simulink subsystem "KF_gyrostellar"  (R2021a)
settings: Solver=VariableStepAuto  StartTime=0.0  StopTime=10.0  RelTol=1e-3
undefined symbols (not defined in the file): bias_gyro_init, gyro_bias_init, init_align_error, magnitude
libraries: dspmtrx3 x1, sharedtransform x1
settings Model: Creator=Laura  LastModifiedBy=jmher

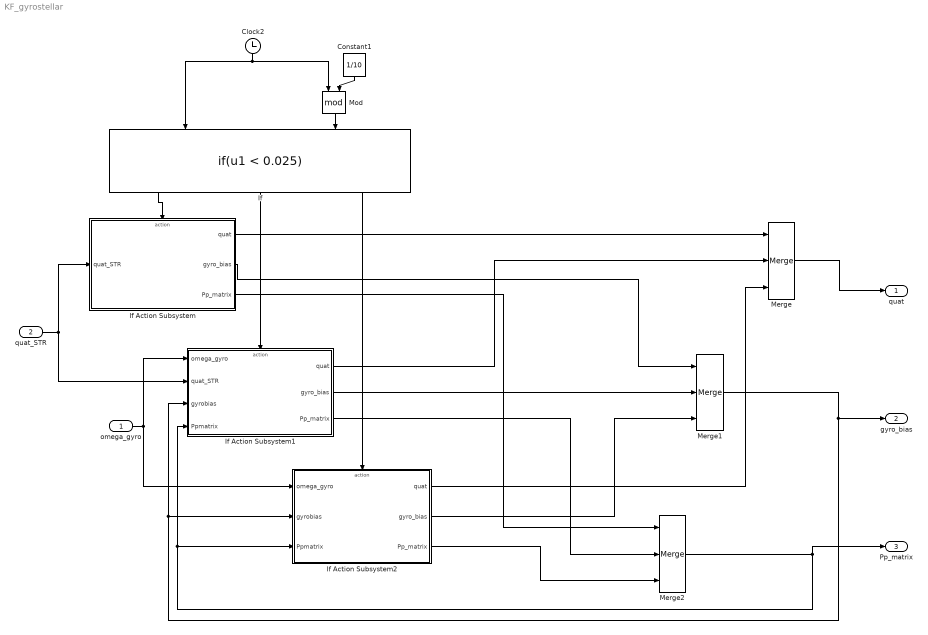
== system KF_gyrostellar ==
  omega_gyro : Inport
  quat_STR : Inport  Port=2
  Clock2 : Clock
  Constant1 : Constant  Value=1/10
  If : If  NumInputs=2  IfExpression=u1 < 0.025  ElseIfExpressions=u2 == 0
  If Action Subsystem : Subsystem  TreatAsAtomicUnit=on
  If Action Subsystem1 : Subsystem  TreatAsAtomicUnit=on
  If Action Subsystem2 : Subsystem  TreatAsAtomicUnit=on
  Merge : Merge  Inputs=3
  Merge1 : Merge  Inputs=3
  Merge2 : Merge  Inputs=3
  Mod : Math  Operator=mod  SaturateOnIntegerOverflow=on
  quat : Outport
  gyro_bias : Outport  Port=2
  Pp_matrix : Outport  Port=3
  wires:
  Clock2/1 -> Mod/1, If/1
  Constant1/1 -> Mod/2
  Mod/1 -> If/2
  If Action Subsystem2/1(quat) -> Merge/3
  Merge/1 -> quat/1
  If Action Subsystem/1(quat) -> Merge/1
  If Action Subsystem/2(gyro_bias) -> Merge1/1
  If Action Subsystem1/2(gyro_bias) -> Merge1/2
  If Action Subsystem2/2(gyro_bias) -> Merge1/3
  If Action Subsystem2/3(Pp_matrix) -> Merge2/3
  If Action Subsystem/3(Pp_matrix) -> Merge2/1
  If Action Subsystem1/3(Pp_matrix) -> Merge2/2
  Merge1/1 -> gyro_bias/1, If Action Subsystem1/3(gyrobias), If Action Subsystem2/2(gyrobias)
  quat_STR/1 -> If Action Subsystem1/2(quat_STR), If Action Subsystem/1(quat_STR)
  Merge2/1 -> Pp_matrix/1, If Action Subsystem2/3(Ppmatrix), If Action Subsystem1/4(Ppmatrix)
  If/1 -> If Action Subsystem/Action
  omega_gyro/1 -> If Action Subsystem2/1(omega_gyro), If Action Subsystem1/1(omega_gyro)
  If/2 -> If Action Subsystem1/Action
  If Action Subsystem1/1(quat) -> Merge/2
  If/3 -> If Action Subsystem2/Action

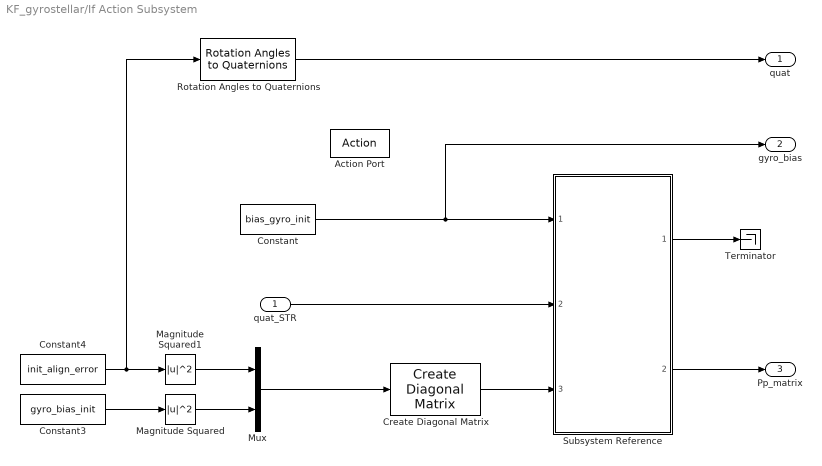
== system KF_gyrostellar/If Action Subsystem ==
  quat_STR : Inport
  Action Port : ActionPort  ActionPortLabel=if(u1 < 0.025)
  Constant : Constant  Value=bias_gyro_init
  Constant3 : Constant  Value=gyro_bias_init
  Constant4 : Constant  Value=init_align_error
  Create Diagonal Matrix : dspmtrx3/Create Diagonal Matrix
      settings: SourceProductBaseCode=DS
  Magnitude Squared : Math  Operator=magnitude^2  SaturateOnIntegerOverflow=on
  Magnitude Squared1 : Math  Operator=magnitude^2  SaturateOnIntegerOverflow=on
  Mux : Mux  Inputs=2
  Rotation Angles to Quaternions : sharedtransform/Rotation Angles to Quaternions  rotationOrder=ZYX  aMode=aMode
      settings: SourceProductBaseCode=AE,PW,DR,MT,UV,VE
  Subsystem Reference : Subsystem  ReferencedSubsystem=KF_update
  Terminator : Terminator
  quat : Outport
  gyro_bias : Outport  Port=2
  Pp_matrix : Outport  Port=3
  wires:
  Magnitude Squared1/1 -> Mux/1
  Constant3/1 -> Magnitude Squared/1
  Mux/1 -> Create Diagonal Matrix/1
  Constant/1 -> gyro_bias/1, Subsystem Reference/1
  Create Diagonal Matrix/1 -> Subsystem Reference/3
  Subsystem Reference/2 -> Pp_matrix/1
  Rotation Angles to Quaternions/1 -> quat/1
  Constant4/1 -> Rotation Angles to Quaternions/1, Magnitude Squared1/1
  Magnitude Squared/1 -> Mux/2
  Subsystem Reference/1 -> Terminator/1
  quat_STR/1 -> Subsystem Reference/2

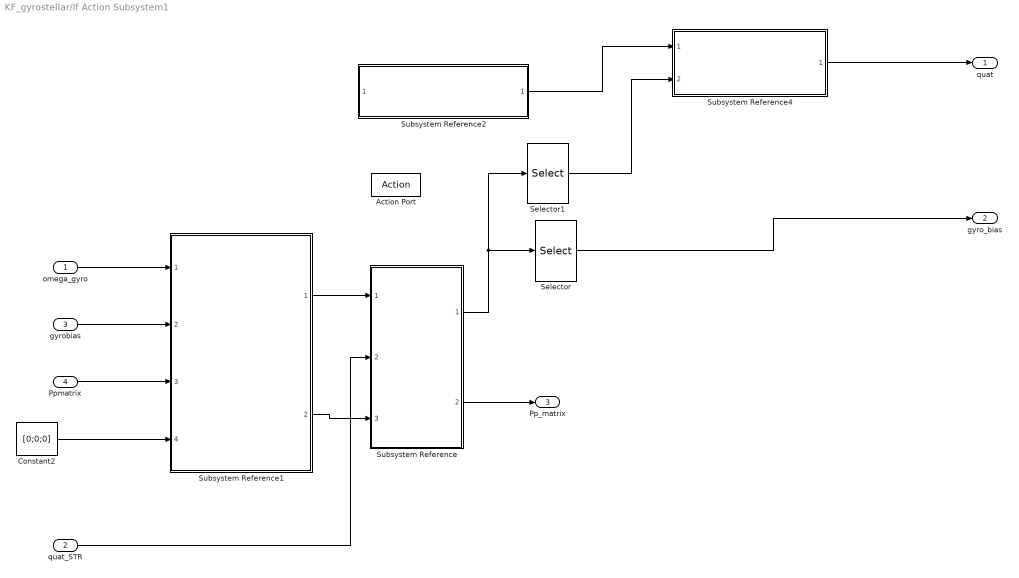
== system KF_gyrostellar/If Action Subsystem1 ==
  omega_gyro : Inport
  quat_STR : Inport  Port=2
  gyrobias : Inport  Port=3
  Ppmatrix : Inport  Port=4
  Action Port : ActionPort  ActionPortLabel=elseif(u2 == 0 )
  Constant2 : Constant  Value=[0;0;0]
  Selector : Selector  InputPortWidth=6  IndexOptions=Index vector (dialog)  Indices=[4 5 6]  OutputSizes=1
  Selector1 : Selector  InputPortWidth=6  IndexOptions=Index vector (dialog)  Indices=[1 2 3]  OutputSizes=1
  Subsystem Reference : Subsystem  ReferencedSubsystem=KF_update
  Subsystem Reference1 : Subsystem  ReferencedSubsystem=KF_prediction
  Subsystem Reference2 : Subsystem  ReferencedSubsystem=GyroIntegrator
  Subsystem Reference4 : Subsystem  ReferencedSubsystem=QuaternionUpdate
  quat : Outport
  gyro_bias : Outport  Port=2
  Pp_matrix : Outport  Port=3
  wires:
  Selector/1 -> gyro_bias/1
  quat_STR/1 -> Subsystem Reference/2
  omega_gyro/1 -> Subsystem Reference1/1
  gyrobias/1 -> Subsystem Reference1/2
  Subsystem Reference/2 -> Pp_matrix/1
  Constant2/1 -> Subsystem Reference1/4
  Subsystem Reference1/1 -> Subsystem Reference/1
  Subsystem Reference4/1 -> quat/1
  Subsystem Reference2/1 -> Subsystem Reference4/1
  Selector1/1 -> Subsystem Reference4/2
  Ppmatrix/1 -> Subsystem Reference1/3
  Subsystem Reference1/2 -> Subsystem Reference/3
  Subsystem Reference/1 -> Selector1/1, Selector/1

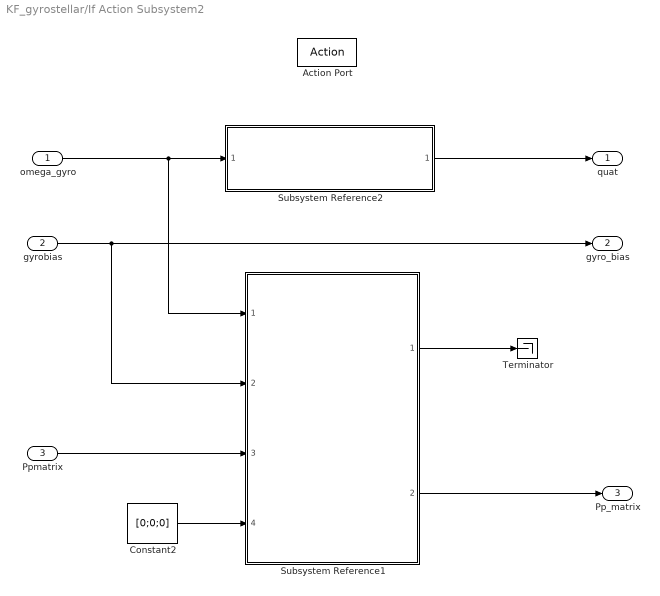
== system KF_gyrostellar/If Action Subsystem2 ==
  omega_gyro : Inport
  gyrobias : Inport  Port=2
  Ppmatrix : Inport  Port=3
  Action Port : ActionPort  ActionPortLabel=else
  Constant2 : Constant  Value=[0;0;0]
  Subsystem Reference1 : Subsystem  ReferencedSubsystem=KF_prediction
  Subsystem Reference2 : Subsystem  ReferencedSubsystem=GyroIntegrator
  Terminator : Terminator
  quat : Outport
  gyro_bias : Outport  Port=2
  Pp_matrix : Outport  Port=3
  wires:
  Subsystem Reference2/1 -> quat/1
  omega_gyro/1 -> Subsystem Reference1/1, Subsystem Reference2/1
  Subsystem Reference1/2 -> Pp_matrix/1
  gyrobias/1 -> Subsystem Reference1/2, gyro_bias/1
  Ppmatrix/1 -> Subsystem Reference1/3
  Constant2/1 -> Subsystem Reference1/4
  Subsystem Reference1/1 -> Terminator/1
